simulink model "demo_modell"  (R2025b)
settings: Solver=VariableStepAuto  StartTime=0.0  StopTime=10.0  RelTol=1e-3
values from neighbouring files (symbols this model uses):
  u1max = 25*pi/180    (= 0.436332312999)    [rcamm.m]
  u1min = -25*pi/180    (= -0.436332312999)    [rcamm.m]
  u2max = 10*pi/180    (= 0.174532925199)    [rcamm.m]
  u2min = -25*pi/180    (= -0.436332312999)    [rcamm.m]
  u3max = 30*pi/180    (= 0.523598775598)    [rcamm.m]
  u3min = - 30*pi/180    (= -0.523598775598)    [rcamm.m]
  u4max = 10*pi/180    (= 0.174532925199)    [rcamm.m]
  u4min = 0.5*pi/180    (= 0.00872664625997)    [rcamm.m]
  u5max = 10*pi/180    (= 0.174532925199)    [rcamm.m]
  u5min = 0.5*pi/180    (= 0.00872664625997)    [rcamm.m]
  Uo = [ ... (first row only)    [linearise.m]
  x0 = [0 ... (first row only)    [initialiseGEODETIC.m]
undefined symbols (not defined in the file or in its folder): RCAM_model_new
libraries: aerolibanimutils x2, aerolibfltsims x1
settings Model: Creator=smthejaswini  LastModifiedBy=smthejaswini

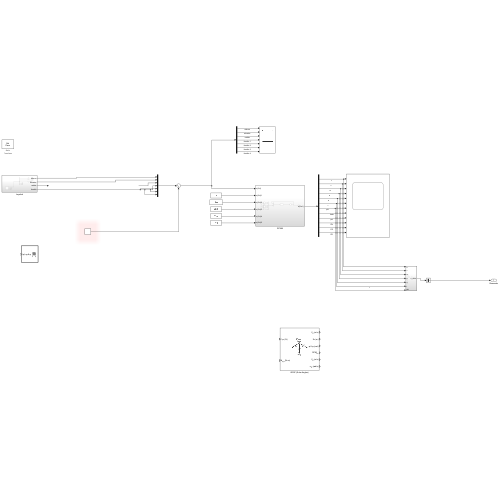
[thumbnail: Simulink's stored preview of the top-level diagram]
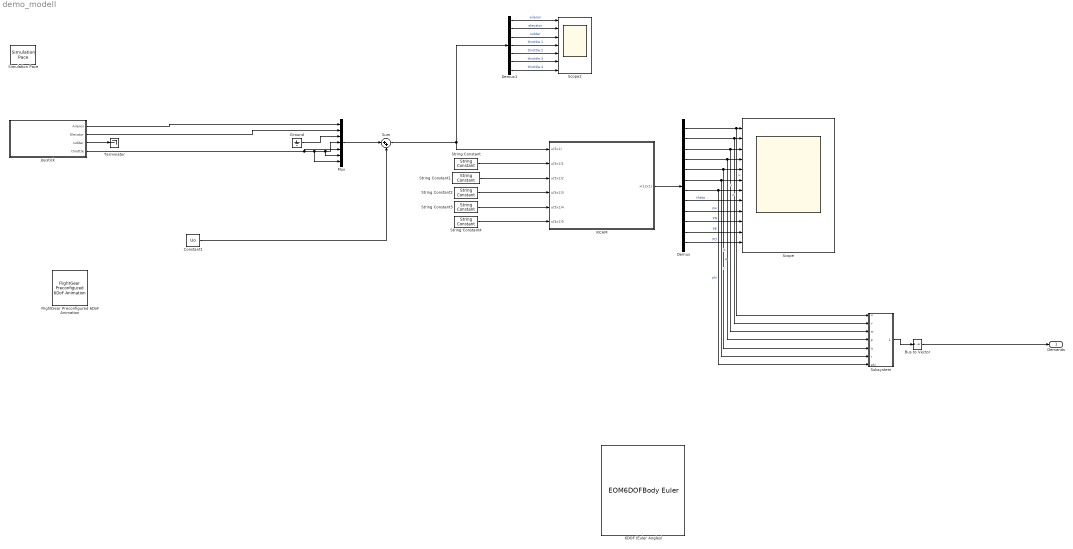
== system demo_modell ==
  6DOF (Euler Angles) : EOM6DOFBodyEuler
  Bus to Vector : BusToVector
  Constant1 : Constant  Value=Uo
  Demux : Demux  Outputs=12
  Demux1 : Demux  Outputs=7
  FlightGear Preconfigured 6DoF Animation : aerolibfltsims/FlightGear Preconfigured 6DoF Animation  xFlightGearVersion=v2019.1  DestinationIpAddress=127.0.0.1  DestinationPort=5502  SampleTime=1/30  packetVersion=24
  Ground : Ground
  Joystick : Subsystem
  Mux : Mux  Inputs=7
  RCAM : Subsystem
  Scope : Scope  NumInputPorts=12
  Scope2 : Scope  NumInputPorts=7
  Simulation Pace : aerolibanimutils/Simulation Pace  SimulationPace=1  SleepMode=Auto  OutputPaceError=off  SampleTime=1/30
  String Constant : StringConstant  String=g
  String Constant1 : StringConstant  String=rho
  String Constant2 : StringConstant  String=Xcg
  String Constant3 : StringConstant  String=Ycg
  String Constant4 : StringConstant  String=Zcg
  Subsystem : Subsystem
  Sum : Sum  Inputs=|++
  Terminator : Terminator
  Demands : Outport  VectorParamsAs1DForOutWhenUnconnected=off
  wires:
  RCAM/1(x(12x1)) -> Demux/1
  Bus to Vector/1 -> Demands/1
  Demux/7 -> Subsystem/7(phi), Scope/7  "phi"
  Demux/8 -> Scope/8  "theta"
  Demux/1 -> Subsystem/1(u), Scope/1  "u"
  Demux1/4 -> Scope2/4  "throttle 1"
  Joystick/4(throttle) -> Mux/7, Mux/6, Mux/4, Mux/5
  Demux/9 -> Scope/9  "psi"
  Demux/12 -> Scope/12  "PD"
  Ground/1 -> Mux/3
  Demux/2 -> Subsystem/2(v), Scope/2  "v"
  Mux/1 -> Sum/1
  String Constant/1 -> RCAM/2(u(5x1)1)
  Demux/11 -> Scope/11  "PE"
  Demux1/3 -> Scope2/3  "rudder"
  Demux/4 -> Subsystem/4(p), Scope/4  "p"
  Demux1/5 -> Scope2/5  "throttle 2"
  Demux/10 -> Scope/10  "PN"
  Joystick/2(Elevator) -> Mux/2
  Demux/5 -> Subsystem/5(q), Scope/5  "q"
  Demux1/1 -> Scope2/1  "aileron"
  String Constant2/1 -> RCAM/4(u(5x1)3)
  Sum/1 -> Demux1/1, RCAM/1(u(5x1))
  String Constant1/1 -> RCAM/3(u(5x1)2)
  Demux/3 -> Subsystem/3(w), Scope/3  "w"
  Demux/6 -> Subsystem/6(r), Scope/6  "r"
  String Constant3/1 -> RCAM/5(u(5x1)4)
  Joystick/3(rudder) -> Terminator/1
  Constant1/1 -> Sum/2
  Demux1/2 -> Scope2/2  "elevator"
  Joystick/1(Aileron) -> Mux/1
  String Constant4/1 -> RCAM/6(u(5x1)5)
  Demux1/6 -> Scope2/6  "throttle 3"
  Demux1/7 -> Scope2/7  "throttle 4"
  Subsystem/1(u_dem) -> Bus to Vector/1

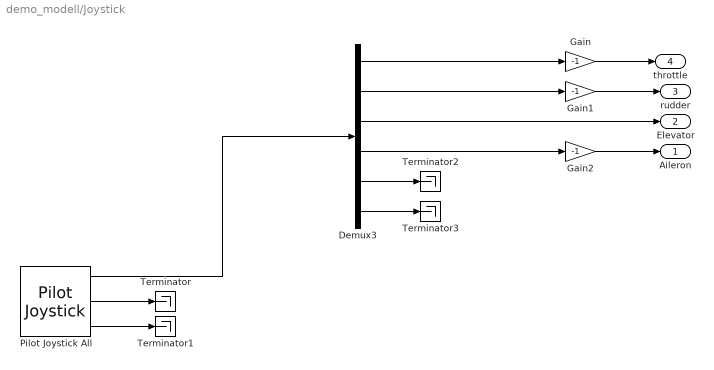
== system demo_modell/Joystick ==
  Demux3 : Demux  Outputs=6
  Gain : Gain  Gain=-1
  Gain1 : Gain  Gain=-1
  Gain2 : Gain  Gain=-1
  Pilot Joystick All : aerolibanimutils/Pilot Joystick  JoystickID=Joystick1  OutputConfiguration=AllOutputs  SampleTime=1/30
      settings: LibrarySourceBlock=aerolibanimutils/Pilot Joystick All
  Terminator{,1..3} (4 alike) : Terminator
  Aileron : Outport
  Elevator : Outport  Port=2
  rudder : Outport  Port=3
  throttle : Outport  Port=4
  wires:
  Demux3/4 -> Gain2/1
  Gain2/1 -> Aileron/1
  Pilot Joystick All/1 -> Demux3/1
  Demux3/2 -> Gain1/1
  Demux3/5 -> Terminator2/1
  Gain1/1 -> rudder/1
  Pilot Joystick All/3 -> Terminator1/1
  Demux3/3 -> Elevator/1
  Gain/1 -> throttle/1
  Pilot Joystick All/2 -> Terminator/1
  Demux3/1 -> Gain/1
  Demux3/6 -> Terminator3/1

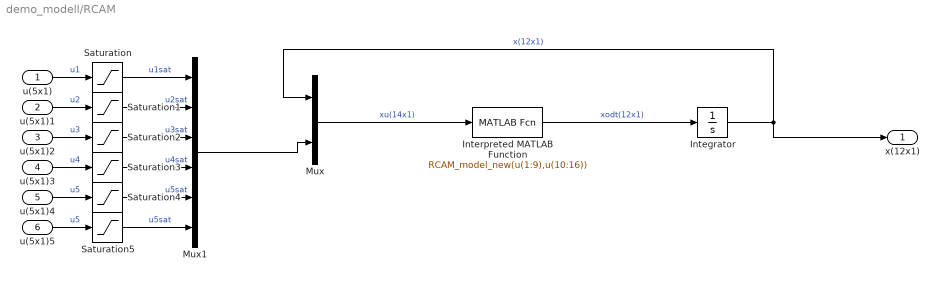
== system demo_modell/RCAM ==
  u(5x1) : Inport
  u(5x1)1 : Inport  Port=2
  u(5x1)2 : Inport  Port=3
  u(5x1)3 : Inport  Port=4
  u(5x1)4 : Inport  Port=5
  u(5x1)5 : Inport  Port=6
  Integrator : Integrator  InitialCondition=x0
  Interpreted MATLAB Function : MATLABFcn  MATLABFcn=RCAM_model_new(u(1:9),u(10:16))
  Mux : Mux  Inputs=2
  Mux1 : Mux  Inputs=6
  Saturation : Saturate  UpperLimit=u1max  LowerLimit=u1min
  Saturation1 : Saturate  UpperLimit=u2max  LowerLimit=u2min
  Saturation2 : Saturate  UpperLimit=u3max  LowerLimit=u3min
  Saturation3 : Saturate  UpperLimit=u4max  LowerLimit=u4min
  Saturation4 : Saturate  UpperLimit=u5max  LowerLimit=u5min
  Saturation5 : Saturate  UpperLimit=u5max  LowerLimit=u5min
  x(12x1) : Outport
  wires:
  Interpreted MATLAB Function/1 -> Integrator/1  "xodt(12x1)"
  Mux/1 -> Interpreted MATLAB Function/1  "xu(14x1)"
  Integrator/1 -> x(12x1)/1, Mux/1  "x(12x1)"
  u(5x1)/1 -> Saturation/1  "u1"
  u(5x1)1/1 -> Saturation1/1  "u2"
  u(5x1)2/1 -> Saturation2/1  "u3"
  u(5x1)3/1 -> Saturation3/1  "u4"
  u(5x1)4/1 -> Saturation4/1  "u5"
  Saturation/1 -> Mux1/1  "u1sat"
  Saturation1/1 -> Mux1/2  "u2sat"
  Saturation2/1 -> Mux1/3  "u3sat"
  Saturation3/1 -> Mux1/4  "u4sat"
  Saturation4/1 -> Mux1/5  "u5sat"
  Mux1/1 -> Mux/2
  u(5x1)5/1 -> Saturation5/1  "u5"
  Saturation5/1 -> Mux1/6  "u5sat"

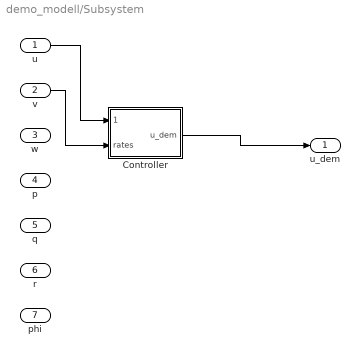
== system demo_modell/Subsystem ==
  u : Inport
  v : Inport  Port=2
  w : Inport  Port=3
  p : Inport  Port=4
  q : Inport  Port=5
  r : Inport  Port=6
  phi : Inport  Port=7
  Controller : MATLAB Function  TreatAsAtomicUnit=on
  u_dem : Outport
  wires:
  u/1 -> Controller/1(demands)
  v/1 -> Controller/2(rates)
  Controller/1(u_dem) -> u_dem/1

== matlab function demo_modell/Subsystem/Controller ==
  data: demands input; u_dem output; rates input
function u_dem = Controller(demands,rates)

Kp = [0.8 0.9 0.5];
Kd = [0.2 0.25 0.15];

roll_cmd  = demands(1);
pitch_cmd = demands(2);
yaw_cmd   = demands(3);

p = rates(1);
q = rates(2);
r = rates(3);

aileron  = Kp(1)*roll_cmd  - Kd(1)*p;
elevator = Kp(2)*pitch_cmd - Kd(2)*q;
rudder   = Kp(3)*yaw_cmd   - Kd(3)*r;

u_dem = zeros(6,1);

u_dem(1) = aileron;
u_dem(2) = elevator;
u_dem(3) = rudder;

end
